simulink model "RxCAN1"  (R2014a)
settings: Solver=ode45  StartTime=0.0  StopTime=10.0  RelTol=1e-3
libraries: simulink x3
settings Model: Creator=10226  LastModifiedBy=10226

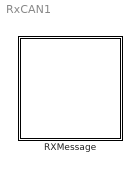
== system RxCAN1 ==
  RXMessage : Subsystem

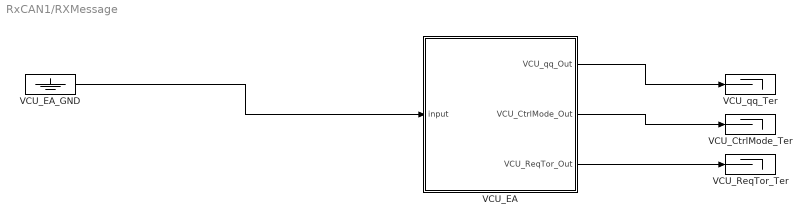
== system RxCAN1/RXMessage ==
  VCU_CtrlMode_Ter : Terminator
  VCU_EA : Subsystem
  VCU_EA_GND : Ground
  VCU_ReqTor_Ter : Terminator
  VCU_qq_Ter : Terminator
  wires:
  VCU_EA/1(VCU_qq_Out) -> VCU_qq_Ter/1
  VCU_EA/2(VCU_CtrlMode_Out) -> VCU_CtrlMode_Ter/1
  VCU_EA/3(VCU_ReqTor_Out) -> VCU_ReqTor_Ter/1
  VCU_EA_GND/1 -> VCU_EA/1(input)

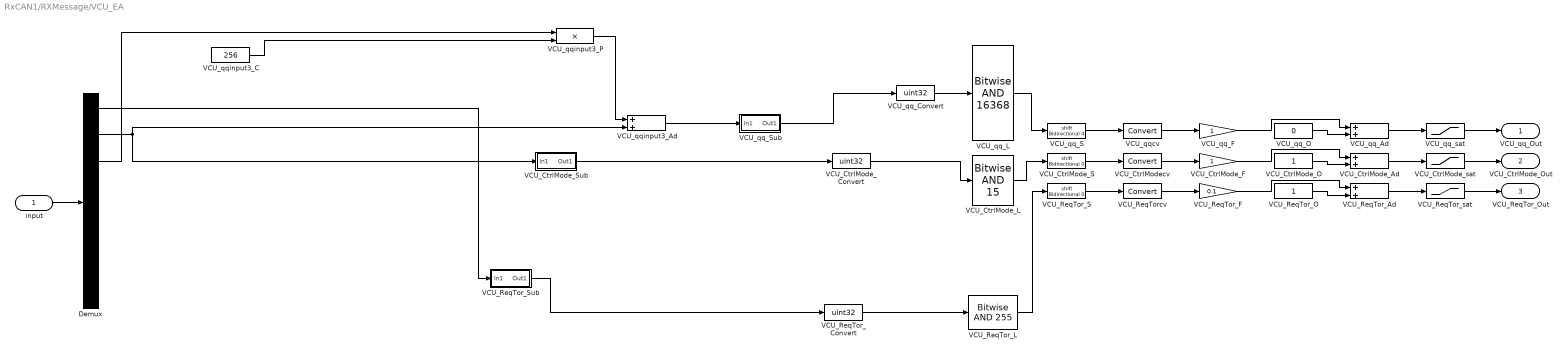
== system RxCAN1/RXMessage/VCU_EA ==
  input : Inport
  Demux : Demux  Outputs=8
  VCU_CtrlMode_Ad : Sum
  VCU_CtrlMode_Convert : DataTypeConversion  OutDataTypeStr=uint32
  VCU_CtrlMode_F : Gain
  VCU_CtrlMode_L : simulink/Logic and Bit Operations/Bitwise Operator  logicop=AND  UseBitMask=on  BitMask=15  BitMaskRealWorld=Stored Integer
  VCU_CtrlMode_O : Constant  OutDataTypeStr=single
  VCU_CtrlMode_S : ArithShift
  VCU_CtrlMode_Sub : Subsystem
  VCU_CtrlMode_sat : Saturate  UpperLimit=16  LowerLimit=1
  VCU_CtrlModecv : DataTypeConversion
  VCU_ReqTor_Ad : Sum
  VCU_ReqTor_Convert : DataTypeConversion  OutDataTypeStr=uint32
  VCU_ReqTor_F : Gain  Gain=0.1
  VCU_ReqTor_L : simulink/Logic and Bit Operations/Bitwise Operator  logicop=AND  UseBitMask=on  BitMask=255  BitMaskRealWorld=Stored Integer
  VCU_ReqTor_O : Constant  OutDataTypeStr=single
  VCU_ReqTor_S : ArithShift
  VCU_ReqTor_Sub : Subsystem
  VCU_ReqTor_sat : Saturate  UpperLimit=26.5  LowerLimit=1
  VCU_ReqTorcv : DataTypeConversion
  VCU_qq_Ad : Sum
  VCU_qq_Convert : DataTypeConversion  OutDataTypeStr=uint32
  VCU_qq_F : Gain
  VCU_qq_L : simulink/Logic and Bit Operations/Bitwise Operator  logicop=AND  UseBitMask=on  BitMask=16368  BitMaskRealWorld=Stored Integer
  VCU_qq_O : Constant  Value=0  OutDataTypeStr=single
  VCU_qq_S : ArithShift  BitShiftNumber=4
  VCU_qq_Sub : Subsystem
  VCU_qq_sat : Saturate  UpperLimit=1023  LowerLimit=0
  VCU_qqcv : DataTypeConversion
  VCU_qqinput3_Ad : Sum
  VCU_qqinput3_C : Constant  Value=256
  VCU_qqinput3_P : Product
  VCU_qq_Out : Outport
  VCU_CtrlMode_Out : Outport  Port=2
  VCU_ReqTor_Out : Outport  Port=3
  wires:
  VCU_qq_F/1 -> VCU_qq_Ad/1
  VCU_qq_O/1 -> VCU_qq_Ad/2
  VCU_qq_Ad/1 -> VCU_qq_sat/1
  VCU_qq_sat/1 -> VCU_qq_Out/1
  Demux/3 -> VCU_qqinput3_P/1
  VCU_qqinput3_C/1 -> VCU_qqinput3_P/2
  VCU_qqinput3_P/1 -> VCU_qqinput3_Ad/1
  Demux/2 -> VCU_qqinput3_Ad/2, VCU_CtrlMode_Sub/1(In1)
  VCU_qqinput3_Ad/1 -> VCU_qq_Sub/1(In1)
  VCU_qq_Sub/1(Out1) -> VCU_qq_Convert/1
  VCU_qq_Convert/1 -> VCU_qq_L/1
  VCU_qq_L/1 -> VCU_qq_S/1
  VCU_qq_S/1 -> VCU_qqcv/1
  VCU_qqcv/1 -> VCU_qq_F/1
  VCU_CtrlMode_F/1 -> VCU_CtrlMode_Ad/1
  VCU_CtrlMode_O/1 -> VCU_CtrlMode_Ad/2
  VCU_CtrlMode_Ad/1 -> VCU_CtrlMode_sat/1
  VCU_CtrlMode_sat/1 -> VCU_CtrlMode_Out/1
  VCU_CtrlMode_Sub/1(Out1) -> VCU_CtrlMode_Convert/1
  VCU_CtrlMode_Convert/1 -> VCU_CtrlMode_L/1
  VCU_CtrlMode_L/1 -> VCU_CtrlMode_S/1
  VCU_CtrlMode_S/1 -> VCU_CtrlModecv/1
  VCU_CtrlModecv/1 -> VCU_CtrlMode_F/1
  VCU_ReqTor_F/1 -> VCU_ReqTor_Ad/1
  VCU_ReqTor_O/1 -> VCU_ReqTor_Ad/2
  VCU_ReqTor_Ad/1 -> VCU_ReqTor_sat/1
  VCU_ReqTor_sat/1 -> VCU_ReqTor_Out/1
  Demux/1 -> VCU_ReqTor_Sub/1(In1)
  VCU_ReqTor_Sub/1(Out1) -> VCU_ReqTor_Convert/1
  VCU_ReqTor_Convert/1 -> VCU_ReqTor_L/1
  VCU_ReqTor_L/1 -> VCU_ReqTor_S/1
  VCU_ReqTor_S/1 -> VCU_ReqTorcv/1
  VCU_ReqTorcv/1 -> VCU_ReqTor_F/1
  input/1 -> Demux/1

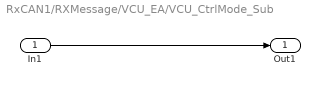
== system RxCAN1/RXMessage/VCU_EA/VCU_CtrlMode_Sub ==
  In1 : Inport
  Out1 : Outport
  wires:
  In1/1 -> Out1/1

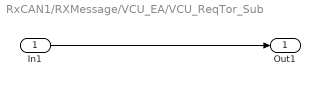
== system RxCAN1/RXMessage/VCU_EA/VCU_ReqTor_Sub ==
  In1 : Inport
  Out1 : Outport
  wires:
  In1/1 -> Out1/1

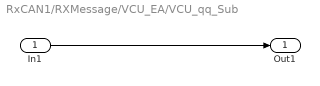
== system RxCAN1/RXMessage/VCU_EA/VCU_qq_Sub ==
  In1 : Inport
  Out1 : Outport
  wires:
  In1/1 -> Out1/1
